simulink model "gm_uz_SVPWM_6ph"  (R2024a)
settings: Solver=FixedStepDiscrete  StartTime=0.0  StopTime=0.0004  RelTol=1e-3
undefined symbols (not defined in the file or in its folder): f_FPGA_clk, T_FPGA_clk
libraries: hdlsllib x7, simulink x1
(part 1 of 2)
settings Model: Creator=josef  LastModifiedBy=josef
settings SolverCC: AlgebraicLoopSolver=TrustRegion
settings DataIOCC: LimitDataPoints=on  SaveOutput=off  SaveTime=off
settings OptimizationCC: BlockReduction=off  ConditionallyExecuteInputs=off  DefaultParameterBehavior=Inlined  LifeSpan=inf
settings DebuggingCC: AlgebraicLoopMsg=error  InheritedTsInSrcMsg=none  SingleTaskRateTransMsg=error  UnconnectedInputMsg=warning  UnconnectedOutputMsg=warning  UnconnectedLineMsg=warning  AllowSymbolicDim=off  StrictBusMsg=ErrorOnBusTreatedAsVector  SFUnexpectedBacktrackingDiag=warning  SFNoUnconditionalDefaultTransitionDiag=warning  SFExecutionAtInitializationDiag=none  ArithmeticOperatorsInVariantConditions=warning
settings HardwareCC: ProdBitPerPointer=32  ProdBitPerSizeT=32  ProdBitPerPtrDiffT=32  ProdLargestAtomicFloat=None  ProdIntDivRoundTo=Undefined  ProdEndianess=Unspecified  ProdWordSize=32  ProdHWDeviceType=ASIC/FPGA->ASIC/FPGA  ProdEqTarget=off
settings ModelReferenceCC: EnableRefExpFcnMdlSchedulingChecks=on
settings SFSimCC: SimUseLocalCustomCode=off  CustomCodeUndefinedFunction=UseInterfaceOnly
settings RTWCC: RTWUseLocalCustomCode=off  GPUComputeCapability=3.5
settings CodeAppCC: StateflowObjectComments=on
settings GRTTargetCC: TargetLangStandard=C89/C90 (ANSI)
settings ConfigComp: CovScope=ReferencedModels  CovMetricSettings=dw  CovSaveCumulativeToWorkspaceVar=on  CovSaveSingleToWorkspaceVar=on  CovExternalEMLEnable=off  CovSFcnEnable=off

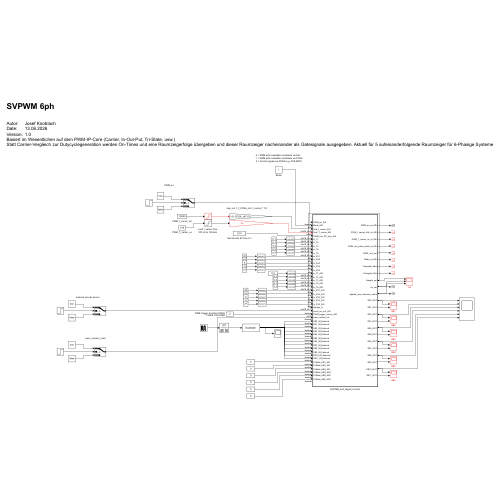
[thumbnail: Simulink's stored preview of the top-level diagram]
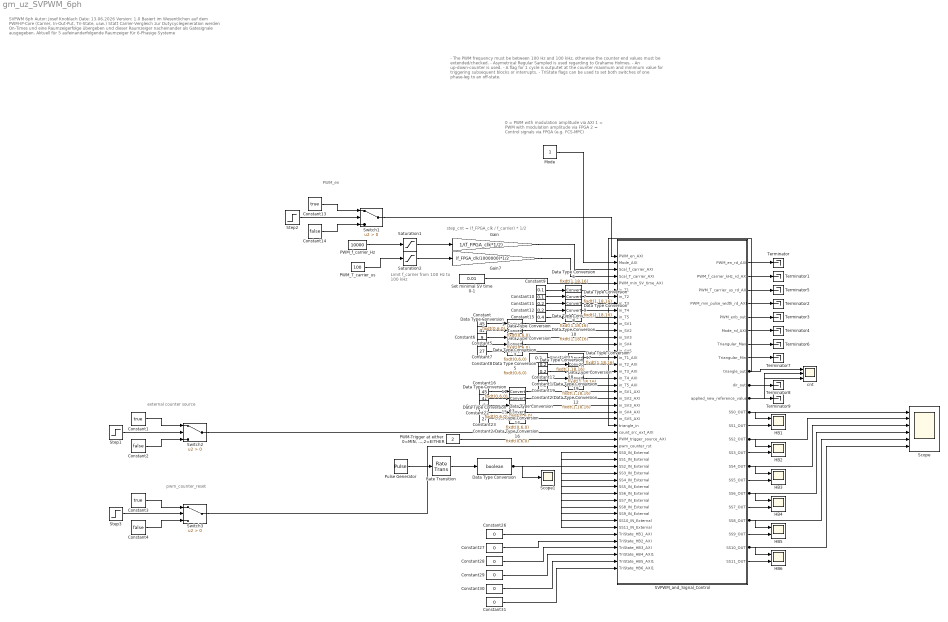
== system gm_uz_SVPWM_6ph ==
  note: pwm_counter_reset
  note: external counter source
  note: 0 = PWM with modulation amplitude via AXI
      | 1 = PWM with modulation amplitude via FPGA
      | 2 = Control signals via FPGA (e.g. FCS-MPC)
  note: step_cnt = (f_FPGA_clk / f_carrier) * 1/2
  note: SVPWM 6ph
      |
      | Autor: Josef Knoblach
      | Date: 13.06.2026
      | Version: 1.0
      | Basiert im Wesentlichen auf dem PWM-IP-Core (Carrier, In-Out-Put, Tri-State, usw.)
      | Statt Carrier-Vergleich zur Dutycyclegeneration werden On-Times und eine Raumzeigerfolge übergeben und dieser Raumzeiger nacheinander als Gatesignale ausgegeben. Aktuell für 5 aufeinanderfolgende Raumzeiger für 6-Phasige Systeme
  note: - The PWM frequency must be between 100 Hz and 100 kHz, otherwise the counter end values must be extended/checked.
      | - Asymetrical Regular Sampled is used regarding to Grahame Holmes.
      | - An up-down-counter is used.
      | - A flag for 1 cycle is outputet at the counter maximum and minimum value for triggering subsequent blocks or interrupts.
      | - TriState flags can be used to set both switches of one phase-leg to an off-state.
  note: Limit f_carrier from
      | 100 Hz to 100 kHz
  note: PWM_en
  Constant : Constant  Value=45  SampleTime=T_FPGA_clk
  Constant1 : Constant  Value=true  SampleTime=T_FPGA_clk
  Constant10 : Constant  Value=0.1  SampleTime=T_FPGA_clk
  Constant{11..12,17..18,20} (5 alike) : Constant  Value=0.2  SampleTime=T_FPGA_clk
  Constant13 : Constant  Value=true  SampleTime=T_FPGA_clk
  Constant14 : Constant  Value=false  SampleTime=T_FPGA_clk
  Constant15 : Constant  Value=0.4  SampleTime=T_FPGA_clk
  Constant16 : Constant  Value=45  SampleTime=T_FPGA_clk
  Constant19 : Constant  Value=0.1  SampleTime=T_FPGA_clk
  Constant2 : Constant  Value=false  SampleTime=T_FPGA_clk
  Constant21 : Constant  Value=41  SampleTime=T_FPGA_clk
  Constant22 : Constant  Value=9  SampleTime=T_FPGA_clk
  Constant23 : Constant  Value=11  SampleTime=T_FPGA_clk
  Constant24 : Constant  Value=27  SampleTime=T_FPGA_clk
  Constant25 : Constant  Value=0.3  SampleTime=T_FPGA_clk
  Constant{26..31} (6 alike) : Constant  Value=0  OutDataTypeStr=boolean  SampleTime=T_FPGA_clk
  Constant3 : Constant  Value=true  SampleTime=T_FPGA_clk
  Constant4 : Constant  Value=false  SampleTime=T_FPGA_clk
  Constant5 : Constant  Value=41  SampleTime=T_FPGA_clk
  Constant6 : Constant  Value=9  SampleTime=T_FPGA_clk
  Constant7 : Constant  Value=11  SampleTime=T_FPGA_clk
  Constant8 : Constant  Value=27  SampleTime=T_FPGA_clk
  Constant9 : Constant  Value=0.1  SampleTime=T_FPGA_clk
  Data Type Conversion : DataTypeConversion  OutDataTypeStr=boolean  SaturateOnIntegerOverflow=off  RndMeth=Floor
  Data Type Conversion{1..5,11,13..16} (10 alike) : DataTypeConversion  OutDataTypeStr=fixdt(0,6,0)  SaturateOnIntegerOverflow=off  RndMeth=Floor
  Data Type Conversion{6..10,12,17..20} (10 alike) : DataTypeConversion  OutDataTypeStr=fixdt(1,18,16)  SaturateOnIntegerOverflow=off  RndMeth=Floor
  Gain : Gain  Gain=1/(f_FPGA_clk*1/2)  OutDataTypeStr=fixdt(0,25,26)
  Gain7 : Gain  Gain=(f_FPGA_clk/1000000)*1/2  OutDataTypeStr=fixdt(0,25,0)
  HB{1..6} (6 alike) : Scope  NumInputPorts=2
  Mode : Constant  OutDataTypeStr=fixdt(0,2,0)  SampleTime=T_FPGA_clk
  "PWM-Trigger at either 0=MIN, 1=MAX,2=EITHER" : Constant  Value=2  OutDataTypeStr=uint32  SampleTime=T_FPGA_clk
  PWM_T_carrier_us : Constant  Value=100  OutDataTypeStr=uint32  SampleTime=T_FPGA_clk
  PWM_f_carrier_Hz : Constant  Value=10000  OutDataTypeStr=uint32  SampleTime=T_FPGA_clk
  Pulse Generator : DiscretePulseGenerator  PulseType=Time based  Period=0.0001  PulseWidth=5
  Rate Transition : RateTransition  OutPortSampleTime=T_FPGA_clk
  SVPWM_and_Signal_Control : Subsystem  TreatAsAtomicUnit=on
  Saturation1 : Saturate  UpperLimit=100000  LowerLimit=100
  Saturation2 : Saturate  UpperLimit=10000  LowerLimit=10
  Scope : Scope  NumInputPorts=6
  Scope1 : Scope
  Set minimal SV time 0-1 : Constant  Value=0.01  OutDataTypeStr=fixdt(1,18,16)  SampleTime=T_FPGA_clk
  Step1 : Step  Time=0.002  After=0  SampleTime=T_FPGA_clk
  Step2 : Step  Time=0.002  Before=1  SampleTime=T_FPGA_clk
  Step3 : Step  Time=0.00025  SampleTime=T_FPGA_clk
  Switch1 : Switch  Criteria=u2 > Threshold  SaturateOnIntegerOverflow=off  InputSameDT=off
  Switch2 : Switch  Criteria=u2 > Threshold  SaturateOnIntegerOverflow=off  InputSameDT=off
  Switch3 : Switch  Criteria=u2 > Threshold  SaturateOnIntegerOverflow=off  InputSameDT=off
  Terminator{,1..9} (10 alike) : Terminator
  cnt : Scope  NumInputPorts=3
  wires:
  SVPWM_and_Signal_Control/15(SS3_OUT) -> HB2/2
  SVPWM_and_Signal_Control/17(SS5_OUT) -> HB3/2
  SVPWM_and_Signal_Control/19(SS7_OUT) -> HB4/2
  SVPWM_and_Signal_Control/21(SS9_OUT) -> HB5/2
  SVPWM_and_Signal_Control/23(SS11_OUT) -> HB6/2
  SVPWM_and_Signal_Control/13(SS1_OUT) -> HB1/2
  SVPWM_and_Signal_Control/22(SS10_OUT) -> Scope/6, HB6/1
  SVPWM_and_Signal_Control/20(SS8_OUT) -> Scope/5, HB5/1
  SVPWM_and_Signal_Control/18(SS6_OUT) -> Scope/4, HB4/1
  SVPWM_and_Signal_Control/16(SS4_OUT) -> Scope/3, HB3/1
  SVPWM_and_Signal_Control/14(SS2_OUT) -> Scope/2, HB2/1
  SVPWM_and_Signal_Control/12(SS0_OUT) -> Scope/1, HB1/1
  Constant31/1 -> SVPWM_and_Signal_Control/47(TriState_HB6_AXI1)
  Constant30/1 -> SVPWM_and_Signal_Control/46(TriState_HB5_AXI1)
  Constant29/1 -> SVPWM_and_Signal_Control/45(TriState_HB4_AXI1)
  Constant28/1 -> SVPWM_and_Signal_Control/44(TriState_HB3_AXI)
  Constant27/1 -> SVPWM_and_Signal_Control/43(TriState_HB2_AXI)
  Constant26/1 -> SVPWM_and_Signal_Control/42(TriState_HB1_AXI)
  Data Type Conversion/1 -> SVPWM_and_Signal_Control/30(SS0_IN_External), SVPWM_and_Signal_Control/31(SS1_IN_External), SVPWM_and_Signal_Control/32(SS2_IN_External), SVPWM_and_Signal_Control/33(SS3_IN_External), SVPWM_and_Signal_Control/34(SS4_IN_External), SVPWM_and_Signal_Control/35(SS5_IN_External), SVPWM_and_Signal_Control/36(SS6_IN_External), SVPWM_and_Signal_Control/37(SS7_IN_External), SVPWM_and_Signal_Control/38(SS8_IN_External), SVPWM_and_Signal_Control/39(SS9_IN_External), SVPWM_and_Signal_Control/40(SS10_IN_External), SVPWM_and_Signal_Control/41(SS11_IN_External), Scope1/1
  Data Type Conversion16/1 -> SVPWM_and_Signal_Control/25(in_SV5_AXI)
  Data Type Conversion15/1 -> SVPWM_and_Signal_Control/24(in_SV4_AXI)
  Data Type Conversion14/1 -> SVPWM_and_Signal_Control/23(in_SV3_AXI)
  Data Type Conversion13/1 -> SVPWM_and_Signal_Control/22(in_SV2_AXI)
  Data Type Conversion11/1 -> SVPWM_and_Signal_Control/21(in_SV1_AXI)
  Constant16/1 -> Data Type Conversion11/1
  Constant24/1 -> Data Type Conversion16/1
  Constant23/1 -> Data Type Conversion15/1
  Constant22/1 -> Data Type Conversion14/1
  Constant21/1 -> Data Type Conversion13/1
  Constant17/1 -> Data Type Conversion18/1
  Constant18/1 -> Data Type Conversion19/1
  Constant19/1 -> Data Type Conversion20/1
  Constant20/1 -> Data Type Conversion12/1
  Constant25/1 -> Data Type Conversion17/1
  Data Type Conversion17/1 -> SVPWM_and_Signal_Control/16(in_T1_AXI)
  Data Type Conversion12/1 -> SVPWM_and_Signal_Control/20(in_T5_AXI)
  Data Type Conversion20/1 -> SVPWM_and_Signal_Control/19(in_T4_AXI)
  Data Type Conversion19/1 -> SVPWM_and_Signal_Control/18(in_T3_AXI)
  Data Type Conversion18/1 -> SVPWM_and_Signal_Control/17(in_T2_AXI)
  Data Type Conversion7/1 -> SVPWM_and_Signal_Control/7(in_T2)
  Data Type Conversion8/1 -> SVPWM_and_Signal_Control/8(in_T3)
  Data Type Conversion9/1 -> SVPWM_and_Signal_Control/9(in_T4)
  Data Type Conversion10/1 -> SVPWM_and_Signal_Control/10(in_T5)
  Data Type Conversion6/1 -> SVPWM_and_Signal_Control/6(in_T1)
  Constant9/1 -> Data Type Conversion6/1
  Constant15/1 -> Data Type Conversion10/1
  Constant12/1 -> Data Type Conversion9/1
  Constant11/1 -> Data Type Conversion8/1
  Constant10/1 -> Data Type Conversion7/1
  Constant5/1 -> Data Type Conversion2/1
  Constant6/1 -> Data Type Conversion3/1
  Constant7/1 -> Data Type Conversion4/1
  Constant8/1 -> Data Type Conversion5/1
  Constant/1 -> Data Type Conversion1/1
  Data Type Conversion1/1 -> SVPWM_and_Signal_Control/11(in_SV1)
  Data Type Conversion2/1 -> SVPWM_and_Signal_Control/12(in_SV2)
  Data Type Conversion3/1 -> SVPWM_and_Signal_Control/13(in_SV3)
  Data Type Conversion4/1 -> SVPWM_and_Signal_Control/14(in_SV4)
  Data Type Conversion5/1 -> SVPWM_and_Signal_Control/15(in_SV5)
  Constant13/1 -> Switch1/1
  PWM_f_carrier_Hz/1 -> Saturation1/1
  Mode/1 -> SVPWM_and_Signal_Control/2(Mode_AXI)
  Set minimal SV time 0-1/1 -> SVPWM_and_Signal_Control/5(PWM_min_SV_time_AXI)
  Step2/1 -> Switch1/2
  SVPWM_and_Signal_Control/8(Triangular_Min) -> Terminator7/1
  Gain/1 -> SVPWM_and_Signal_Control/3(Scal_f_carrier_AXI)
  SVPWM_and_Signal_Control/6(Mode_rd_AXI) -> Terminator4/1
  Gain7/1 -> SVPWM_and_Signal_Control/4(Scal_T_carrier_AXI)
  SVPWM_and_Signal_Control/5(PWM_enb_out) -> Terminator3/1
  SVPWM_and_Signal_Control/2(PWM_f_carrier_kHz_rd_AXI) -> Terminator1/1
  SVPWM_and_Signal_Control/7(Triangular_Max) -> Terminator6/1
  Constant1/1 -> Switch2/1
  SVPWM_and_Signal_Control/10(dir_out) -> Terminator8/1, cnt/2
  Constant14/1 -> Switch1/3
  Constant2/1 -> Switch2/3
  Saturation1/1 -> Gain/1
  Saturation2/1 -> Gain7/1
  Step1/1 -> Switch2/2
  PWM_T_carrier_us/1 -> Saturation2/1
  Rate Transition/1 -> Data Type Conversion/1
  SVPWM_and_Signal_Control/4(PWM_min_pulse_width_rd_AXI) -> Terminator2/1
  Switch2/1 -> SVPWM_and_Signal_Control/27(count_src_ext_AXI)
  Switch3/1 -> SVPWM_and_Signal_Control/29(pwm_counter_rst)
  SVPWM_and_Signal_Control/3(PWM_T_carrier_us_rd_AXI) -> Terminator5/1
  "PWM-Trigger at either 0=MIN, 1=MAX,2=EITHER"/1 -> SVPWM_and_Signal_Control/28(PWM_trigger_source_AXI)
  Step3/1 -> Switch3/2
  SVPWM_and_Signal_Control/1(PWM_en_rd_AXI) -> Terminator/1
  Switch1/1 -> SVPWM_and_Signal_Control/1(PWM_en_AXI)
  Constant4/1 -> Switch3/3
  SVPWM_and_Signal_Control/11(applied_new_reference_value) -> Terminator9/1, cnt/3
  Pulse Generator/1 -> Rate Transition/1
  Constant3/1 -> Switch3/1
  SVPWM_and_Signal_Control/9(triangle_out) -> cnt/1, SVPWM_and_Signal_Control/26(triangle_in)

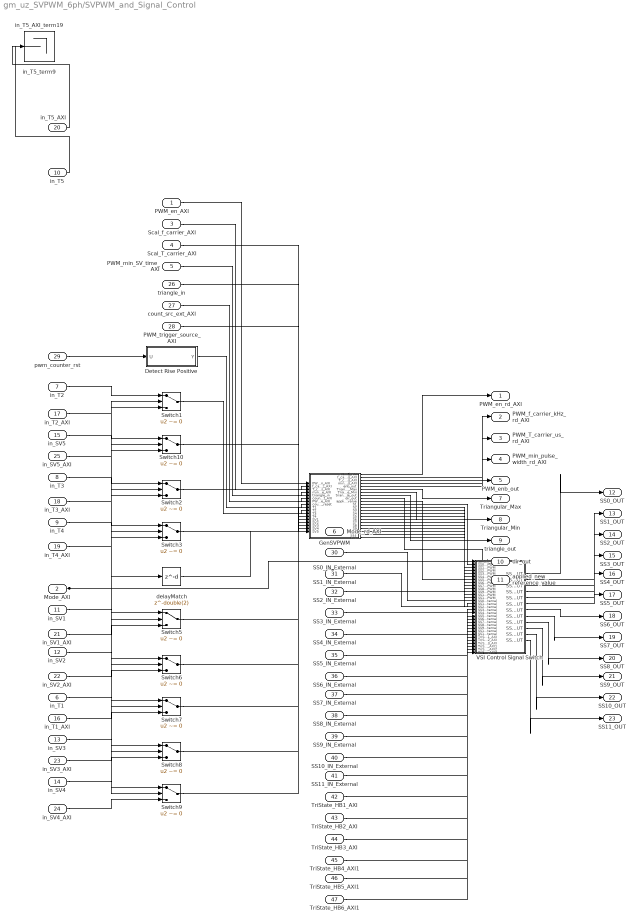
== system gm_uz_SVPWM_6ph/SVPWM_and_Signal_Control ==
  PWM_en_AXI : Inport  OutDataTypeStr=boolean  PortDimensions=1  SampleTime=1e-08
  Mode_AXI : Inport  Port=2  OutDataTypeStr=fixdt(0, 2, 0)  PortDimensions=1  SampleTime=1e-08
  Scal_f_carrier_AXI : Inport  Port=3  OutDataTypeStr=fixdt(0, 25, 26)  PortDimensions=1  SampleTime=1e-08
  Scal_T_carrier_AXI : Inport  Port=4  OutDataTypeStr=fixdt(0, 25, 0)  PortDimensions=1  SampleTime=1e-08
  PWM_min_SV_time_AXI : Inport  Port=5  OutDataTypeStr=fixdt(1, 18, 16)  PortDimensions=1  SampleTime=1e-08
  in_T1 : Inport  Port=6  OutDataTypeStr=fixdt(1, 18, 16)  PortDimensions=1  SampleTime=1e-08
  in_T2 : Inport  Port=7  OutDataTypeStr=fixdt(1, 18, 16)  PortDimensions=1  SampleTime=1e-08
  in_T3 : Inport  Port=8  OutDataTypeStr=fixdt(1, 18, 16)  PortDimensions=1  SampleTime=1e-08
  in_T4 : Inport  Port=9  OutDataTypeStr=fixdt(1, 18, 16)  PortDimensions=1  SampleTime=1e-08
  in_T5 : Inport  Port=10  OutDataTypeStr=fixdt(1, 18, 16)  PortDimensions=1  SampleTime=1e-08
  in_SV1 : Inport  Port=11  OutDataTypeStr=fixdt(0, 6, 0)  PortDimensions=1  SampleTime=1e-08
  in_SV2 : Inport  Port=12  OutDataTypeStr=fixdt(0, 6, 0)  PortDimensions=1  SampleTime=1e-08
  in_SV3 : Inport  Port=13  OutDataTypeStr=fixdt(0, 6, 0)  PortDimensions=1  SampleTime=1e-08
  in_SV4 : Inport  Port=14  OutDataTypeStr=fixdt(0, 6, 0)  PortDimensions=1  SampleTime=1e-08
  in_SV5 : Inport  Port=15  OutDataTypeStr=fixdt(0, 6, 0)  PortDimensions=1  SampleTime=1e-08
  in_T1_AXI : Inport  Port=16  OutDataTypeStr=fixdt(1, 18, 16)  PortDimensions=1  SampleTime=1e-08
  in_T2_AXI : Inport  Port=17  OutDataTypeStr=fixdt(1, 18, 16)  PortDimensions=1  SampleTime=1e-08
  in_T3_AXI : Inport  Port=18  OutDataTypeStr=fixdt(1, 18, 16)  PortDimensions=1  SampleTime=1e-08
  in_T4_AXI : Inport  Port=19  OutDataTypeStr=fixdt(1, 18, 16)  PortDimensions=1  SampleTime=1e-08
  in_T5_AXI : Inport  Port=20  OutDataTypeStr=fixdt(1, 18, 16)  PortDimensions=1  SampleTime=1e-08
  in_SV1_AXI : Inport  Port=21  OutDataTypeStr=fixdt(0, 6, 0)  PortDimensions=1  SampleTime=1e-08
  in_SV2_AXI : Inport  Port=22  OutDataTypeStr=fixdt(0, 6, 0)  PortDimensions=1  SampleTime=1e-08
  in_SV3_AXI : Inport  Port=23  OutDataTypeStr=fixdt(0, 6, 0)  PortDimensions=1  SampleTime=1e-08
  in_SV4_AXI : Inport  Port=24  OutDataTypeStr=fixdt(0, 6, 0)  PortDimensions=1  SampleTime=1e-08
  in_SV5_AXI : Inport  Port=25  OutDataTypeStr=fixdt(0, 6, 0)  PortDimensions=1  SampleTime=1e-08
  triangle_in : Inport  Port=26  OutDataTypeStr=fixdt(0, 18, 17)  PortDimensions=1  SampleTime=1e-08
  count_src_ext_AXI : Inport  Port=27  OutDataTypeStr=boolean  PortDimensions=1  SampleTime=1e-08
  PWM_trigger_source_AXI : Inport  Port=28  OutDataTypeStr=uint32  PortDimensions=1  SampleTime=1e-08
  pwm_counter_rst : Inport  Port=29  OutDataTypeStr=boolean  PortDimensions=1  SampleTime=1e-08
  SS0_IN_External : Inport  Port=30  OutDataTypeStr=boolean  PortDimensions=1  SampleTime=1e-08
  SS1_IN_External : Inport  Port=31  OutDataTypeStr=boolean  PortDimensions=1  SampleTime=1e-08
  SS2_IN_External : Inport  Port=32  OutDataTypeStr=boolean  PortDimensions=1  SampleTime=1e-08
  SS3_IN_External : Inport  Port=33  OutDataTypeStr=boolean  PortDimensions=1  SampleTime=1e-08
  SS4_IN_External : Inport  Port=34  OutDataTypeStr=boolean  PortDimensions=1  SampleTime=1e-08
  SS5_IN_External : Inport  Port=35  OutDataTypeStr=boolean  PortDimensions=1  SampleTime=1e-08
  SS6_IN_External : Inport  Port=36  OutDataTypeStr=boolean  PortDimensions=1  SampleTime=1e-08
  SS7_IN_External : Inport  Port=37  OutDataTypeStr=boolean  PortDimensions=1  SampleTime=1e-08
  SS8_IN_External : Inport  Port=38  OutDataTypeStr=boolean  PortDimensions=1  SampleTime=1e-08
  SS9_IN_External : Inport  Port=39  OutDataTypeStr=boolean  PortDimensions=1  SampleTime=1e-08
  SS10_IN_External : Inport  Port=40  OutDataTypeStr=boolean  PortDimensions=1  SampleTime=1e-08
  SS11_IN_External : Inport  Port=41  OutDataTypeStr=boolean  PortDimensions=1  SampleTime=1e-08
  TriState_HB1_AXI : Inport  Port=42  OutDataTypeStr=boolean  PortDimensions=1  SampleTime=1e-08
  TriState_HB2_AXI : Inport  Port=43  OutDataTypeStr=boolean  PortDimensions=1  SampleTime=1e-08
  TriState_HB3_AXI : Inport  Port=44  OutDataTypeStr=boolean  PortDimensions=1  SampleTime=1e-08
  TriState_HB4_AXI1 : Inport  Port=45  OutDataTypeStr=boolean  PortDimensions=1  SampleTime=1e-08
  TriState_HB5_AXI1 : Inport  Port=46  OutDataTypeStr=boolean  PortDimensions=1  SampleTime=1e-08
  TriState_HB6_AXI1 : Inport  Port=47  OutDataTypeStr=boolean  PortDimensions=1  SampleTime=1e-08
  Detect Rise Positive : Subsystem  mask(Detect Rise Positive){vinit=double(0), InputProcessing=Elements as channels (sample based), OutDataTypeStr=boolean}
      mask prompts: vinit "Simulink:masks:InitialCondition_MP"; InputProcessing "Simulink:masks:InputProcessing_MP"; OutDataTypeStr "Simulink:masks:OutputDataType_MP"
      mask help: Simulink:masks:DetectRisePositive_MD
      mask init:
      | InputProcessing = 'Elements as channels (sample based)';
      | OutDataTypeStr = 'boolean';
      | vinit = double(0);
      mask TypeOptions InputProcessing: Simulink:masks:ColumnsAsChannelsFrameBased | Simulink:masks:ElementsAsChannelsSampleBased
      mask TypeOptions OutDataTypeStr: Simulink:masks:uint8 | Simulink:masks:boolean
      mask Display: fprintf('U > 0\n&  NOT\nU/z > 0')
  GenSVPWM : Subsystem
  Switch{1..3,7} (4 alike) : Switch  Criteria=u2 ~= 0  Threshold=double(0)  OutDataTypeStr=fixdt(1, 18, 16)  SampleTime=1e-08  SaturateOnIntegerOverflow=off  InputSameDT=off
  Switch{5..6,8..10} (5 alike) : Switch  Criteria=u2 ~= 0  Threshold=double(0)  OutDataTypeStr=fixdt(0, 6, 0)  SampleTime=1e-08  SaturateOnIntegerOverflow=off  InputSameDT=off
  VSI Control Signal Switch : Subsystem
  delayMatch : Delay  DelayLength=double(2)  InitialCondition=0  SampleTime=1e-08
  in_T5_AXI_term19 : Terminator
  in_T5_term9 : Terminator
  PWM_en_rd_AXI : Outport  SampleTime=1e-08  VectorParamsAs1DForOutWhenUnconnected=off
  PWM_f_carrier_kHz_rd_AXI : Outport  Port=2  SampleTime=1e-08  VectorParamsAs1DForOutWhenUnconnected=off
  PWM_T_carrier_us_rd_AXI : Outport  Port=3  SampleTime=1e-08  VectorParamsAs1DForOutWhenUnconnected=off
  PWM_min_pulse_width_rd_AXI : Outport  Port=4  SampleTime=1e-08  VectorParamsAs1DForOutWhenUnconnected=off
  PWM_enb_out : Outport  Port=5  SampleTime=1e-08  VectorParamsAs1DForOutWhenUnconnected=off
  Mode_rd_AXI : Outport  Port=6  SampleTime=1e-08  VectorParamsAs1DForOutWhenUnconnected=off
  Triangular_Max : Outport  Port=7  SampleTime=1e-08  VectorParamsAs1DForOutWhenUnconnected=off
  Triangular_Min : Outport  Port=8  SampleTime=1e-08  VectorParamsAs1DForOutWhenUnconnected=off
  triangle_out : Outport  Port=9  SampleTime=1e-08  VectorParamsAs1DForOutWhenUnconnected=off
  dir_out : Outport  Port=10  SampleTime=1e-08  VectorParamsAs1DForOutWhenUnconnected=off
  applied_new_reference_value : Outport  Port=11  SampleTime=1e-08  VectorParamsAs1DForOutWhenUnconnected=off
  SS0_OUT : Outport  Port=12  SampleTime=1e-08  VectorParamsAs1DForOutWhenUnconnected=off
  SS1_OUT : Outport  Port=13  SampleTime=1e-08  VectorParamsAs1DForOutWhenUnconnected=off
  SS2_OUT : Outport  Port=14  SampleTime=1e-08  VectorParamsAs1DForOutWhenUnconnected=off
  SS3_OUT : Outport  Port=15  SampleTime=1e-08  VectorParamsAs1DForOutWhenUnconnected=off
  SS4_OUT : Outport  Port=16  SampleTime=1e-08  VectorParamsAs1DForOutWhenUnconnected=off
  SS5_OUT : Outport  Port=17  SampleTime=1e-08  VectorParamsAs1DForOutWhenUnconnected=off
  SS6_OUT : Outport  Port=18  SampleTime=1e-08  VectorParamsAs1DForOutWhenUnconnected=off
  SS7_OUT : Outport  Port=19  SampleTime=1e-08  VectorParamsAs1DForOutWhenUnconnected=off
  SS8_OUT : Outport  Port=20  SampleTime=1e-08  VectorParamsAs1DForOutWhenUnconnected=off
  SS9_OUT : Outport  Port=21  SampleTime=1e-08  VectorParamsAs1DForOutWhenUnconnected=off
  SS10_OUT : Outport  Port=22  SampleTime=1e-08  VectorParamsAs1DForOutWhenUnconnected=off
  SS11_OUT : Outport  Port=23  SampleTime=1e-08  VectorParamsAs1DForOutWhenUnconnected=off
  wires:
  PWM_en_AXI/1 -> GenSVPWM/1(PWM_en_AXI)
  delayMatch/1 -> Mode_rd_AXI/1
  Scal_f_carrier_AXI/1 -> GenSVPWM/2(f_carrier_kHz_AXI)
  Scal_T_carrier_AXI/1 -> GenSVPWM/3(T_carrier_us_AXI)
  PWM_min_SV_time_AXI/1 -> GenSVPWM/4(min_SV_time_AXI)
  in_T1/1 -> Switch7/1
  in_T2/1 -> Switch1/1
  in_T3/1 -> Switch2/1
  in_T4/1 -> Switch3/1
  in_T5/1 -> in_T5_term9/1
  in_SV1/1 -> Switch5/1
  in_SV2/1 -> Switch6/1
  in_SV3/1 -> Switch8/1
  in_SV4/1 -> Switch9/1
  in_SV5/1 -> Switch10/1
  in_T1_AXI/1 -> Switch7/3
  in_T2_AXI/1 -> Switch1/3
  in_T3_AXI/1 -> Switch2/3
  in_T4_AXI/1 -> Switch3/3
  in_T5_AXI/1 -> in_T5_AXI_term19/1
  in_SV1_AXI/1 -> Switch5/3
  in_SV2_AXI/1 -> Switch6/3
  in_SV3_AXI/1 -> Switch8/3
  in_SV4_AXI/1 -> Switch9/3
  in_SV5_AXI/1 -> Switch10/3
  triangle_in/1 -> GenSVPWM/5(triangle_in)
  count_src_ext_AXI/1 -> GenSVPWM/6(count_src_ext_AXI)
  PWM_trigger_source_AXI/1 -> GenSVPWM/7(PWM_trigger_source_AXI)
  pwm_counter_rst/1 -> Detect Rise Positive/1(U)
  SS0_IN_External/1 -> VSI Control Signal Switch/14(SS0_IN_External)
  SS1_IN_External/1 -> VSI Control Signal Switch/15(SS1_IN_External)
  SS2_IN_External/1 -> VSI Control Signal Switch/16(SS2_IN_External)
  SS3_IN_External/1 -> VSI Control Signal Switch/17(SS3_IN_External)
  SS4_IN_External/1 -> VSI Control Signal Switch/18(SS4_IN_External)
  SS5_IN_External/1 -> VSI Control Signal Switch/19(SS5_IN_External)
  SS6_IN_External/1 -> VSI Control Signal Switch/20(SS6_IN_External)
  SS7_IN_External/1 -> VSI Control Signal Switch/21(SS7_IN_External)
  SS8_IN_External/1 -> VSI Control Signal Switch/22(SS8_IN_External)
  SS9_IN_External/1 -> VSI Control Signal Switch/23(SS9_IN_External)
  SS10_IN_External/1 -> VSI Control Signal Switch/24(SS10_IN_External)
  SS11_IN_External/1 -> VSI Control Signal Switch/25(SS11_IN_External)
  TriState_HB1_AXI/1 -> VSI Control Signal Switch/26(TriState_HB1_AXI)
  TriState_HB2_AXI/1 -> VSI Control Signal Switch/27(TriState_HB2_AXI)
  TriState_HB3_AXI/1 -> VSI Control Signal Switch/28(TriState_HB3_AXI)
  TriState_HB4_AXI1/1 -> VSI Control Signal Switch/29(TriState_HB4_AXI1)
  TriState_HB5_AXI1/1 -> VSI Control Signal Switch/30(TriState_HB5_AXI2)
  TriState_HB6_AXI1/1 -> VSI Control Signal Switch/31(TriState_HB6_AXI3)
  Detect Rise Positive/1(Y) -> GenSVPWM/8(counter_reset)
  GenSVPWM/1(PWM_en_rd_AXI) -> PWM_en_rd_AXI/1
  GenSVPWM/2(f_carrier_kHz_rd_AXI) -> PWM_f_carrier_kHz_rd_AXI/1
  GenSVPWM/3(T_carrier_us_rd_AXI) -> PWM_T_carrier_us_rd_AXI/1
  GenSVPWM/4(min_SV_time_rd_AXI) -> PWM_min_pulse_width_rd_AXI/1
  GenSVPWM/5(enb_out) -> PWM_enb_out/1
  GenSVPWM/6(Triangle_Max) -> Triangular_Max/1
  GenSVPWM/7(Triangle_Min) -> Triangular_Min/1
  GenSVPWM/8(triangle_out) -> triangle_out/1
  GenSVPWM/9(dir_out) -> dir_out/1
  GenSVPWM/10(applied_new_reference_value) -> applied_new_reference_value/1
  GenSVPWM/11(S1) -> VSI Control Signal Switch/2(SS0_IN_PWM)
  GenSVPWM/12(S2) -> VSI Control Signal Switch/3(SS1_IN_PWM)
  GenSVPWM/13(S3) -> VSI Control Signal Switch/4(SS2_IN_PWM)
  GenSVPWM/14(S4) -> VSI Control Signal Switch/5(SS3_IN_PWM)
  GenSVPWM/15(S5) -> VSI Control Signal Switch/6(SS4_IN_PWM)
  GenSVPWM/16(S6) -> VSI Control Signal Switch/7(SS5_IN_PWM)
  GenSVPWM/17(S7) -> VSI Control Signal Switch/8(SS6_IN_PWM)
  GenSVPWM/18(S8) -> VSI Control Signal Switch/9(SS7_IN_PWM)
  GenSVPWM/19(S9) -> VSI Control Signal Switch/10(SS8_IN_PWM)
  GenSVPWM/20(S10) -> VSI Control Signal Switch/11(SS9_IN_PWM)
  GenSVPWM/21(S11) -> VSI Control Signal Switch/12(SS10_IN_PWM)
  GenSVPWM/22(S12) -> VSI Control Signal Switch/13(SS11_IN_PWM)
  Switch1/1 -> GenSVPWM/10(T2)
  Switch10/1 -> GenSVPWM/17(SV5)
  Switch2/1 -> GenSVPWM/11(T3)
  Switch3/1 -> GenSVPWM/12(T4)
  Switch5/1 -> GenSVPWM/13(SV1)
  Switch6/1 -> GenSVPWM/14(SV2)
  Switch7/1 -> GenSVPWM/9(T1)
  Switch8/1 -> GenSVPWM/15(SV3)
  Switch9/1 -> GenSVPWM/16(SV4)
  VSI Control Signal Switch/1(SS0_OUT) -> SS0_OUT/1
  VSI Control Signal Switch/2(SS1_OUT) -> SS1_OUT/1
  VSI Control Signal Switch/3(SS2_OUT) -> SS2_OUT/1
  VSI Control Signal Switch/4(SS3_OUT) -> SS3_OUT/1
  VSI Control Signal Switch/5(SS4_OUT) -> SS4_OUT/1
  VSI Control Signal Switch/6(SS5_OUT) -> SS5_OUT/1
  VSI Control Signal Switch/7(SS6_OUT) -> SS6_OUT/1
  VSI Control Signal Switch/8(SS7_OUT) -> SS7_OUT/1
  VSI Control Signal Switch/9(SS8_OUT) -> SS8_OUT/1
  VSI Control Signal Switch/10(SS9_OUT) -> SS9_OUT/1
  VSI Control Signal Switch/11(SS10_OUT) -> SS10_OUT/1
  VSI Control Signal Switch/12(SS11_OUT) -> SS11_OUT/1
  Mode_AXI/1 -> delayMatch/1, Switch9/2, Switch8/2, Switch7/2, Switch6/2, Switch5/2, Switch3/2, Switch2/2, Switch10/2, Switch1/2, VSI Control Signal Switch/1(Switch_AXI)

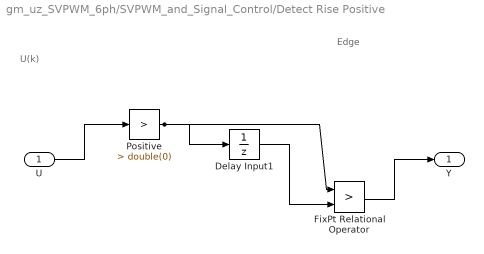
== system gm_uz_SVPWM_6ph/SVPWM_and_Signal_Control/Detect Rise Positive ==
  note: U(k)
  note: Edge
  U : Inport  OutDataTypeStr=boolean  SampleTime=1e-08
  Delay Input1 : UnitDelay  SampleTime=1e-08
  FixPt Relational Operator : RelationalOperator  Operator=>  OutDataTypeStr=boolean  SampleTime=1e-08  InputSameDT=off
  Positive : simulink/Logic and Bit Operations/Compare To Constant  relop=>  const=double(0)  OutDataTypeStr=boolean
  Y : Outport  SampleTime=1e-08
  wires:
  U/1 -> Positive/1
  Delay Input1/1 -> FixPt Relational Operator/2
  FixPt Relational Operator/1 -> Y/1
  Positive/1 -> FixPt Relational Operator/1, Delay Input1/1

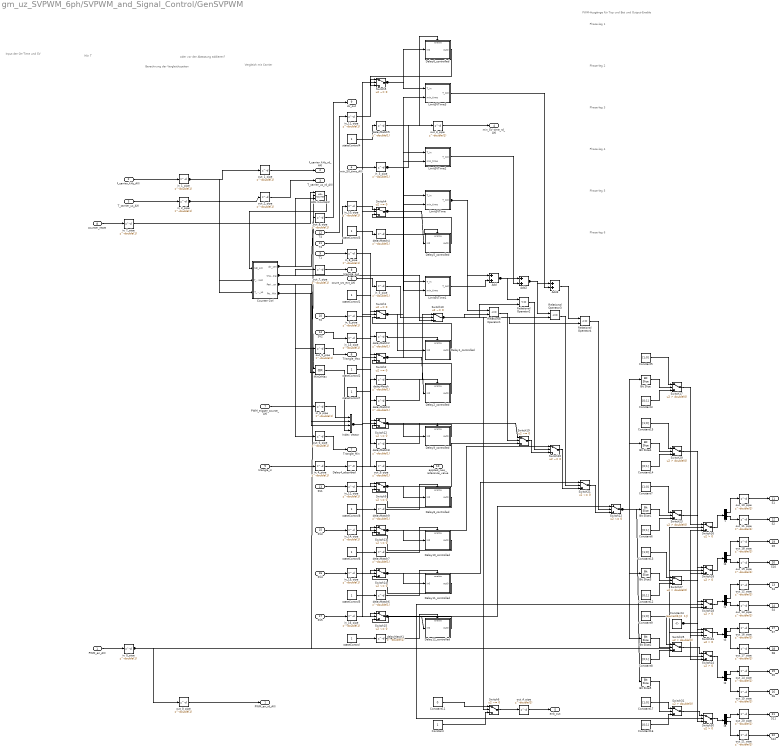
== system gm_uz_SVPWM_6ph/SVPWM_and_Signal_Control/GenSVPWM ==
  note: Phase-leg 6
  note: Phase-leg 5
  note: Phase-leg 4
  note: Phase-leg 3
  note: Phase-leg 2
  note: Phase-leg 1
  note: oder vor der Abtastung addieren?
  note: Input der On-Time und SV
  note: Berechnung der Vergleichszeiten
  note: Vergleich mit Carrier
  note: PWM-Ausgänge für Top und Bot und Output-Enable
  note: Min T
  PWM_en_AXI : Inport  OutDataTypeStr=boolean  PortDimensions=1  SampleTime=1e-08
  f_carrier_kHz_AXI : Inport  Port=2  OutDataTypeStr=fixdt(0, 25, 26)  PortDimensions=1  SampleTime=1e-08
  T_carrier_us_AXI : Inport  Port=3  OutDataTypeStr=fixdt(0, 25, 0)  PortDimensions=1  SampleTime=1e-08
  min_SV_time_AXI : Inport  Port=4  OutDataTypeStr=fixdt(1, 18, 16)  PortDimensions=1  SampleTime=1e-08
  triangle_in : Inport  Port=5  OutDataTypeStr=fixdt(0, 18, 17)  PortDimensions=1  SampleTime=1e-08
  count_src_ext_AXI : Inport  Port=6  OutDataTypeStr=boolean  PortDimensions=1  SampleTime=1e-08
  PWM_trigger_source_AXI : Inport  Port=7  OutDataTypeStr=uint32  PortDimensions=1  SampleTime=1e-08
  counter_reset : Inport  Port=8  OutDataTypeStr=boolean  PortDimensions=1  SampleTime=1e-08
  T1 : Inport  Port=9  OutDataTypeStr=fixdt(1, 18, 16)  PortDimensions=1  SampleTime=1e-08
  T2 : Inport  Port=10  OutDataTypeStr=fixdt(1, 18, 16)  PortDimensions=1  SampleTime=1e-08
  T3 : Inport  Port=11  OutDataTypeStr=fixdt(1, 18, 16)  PortDimensions=1  SampleTime=1e-08
  T4 : Inport  Port=12  OutDataTypeStr=fixdt(1, 18, 16)  PortDimensions=1  SampleTime=1e-08
  SV1 : Inport  Port=13  OutDataTypeStr=fixdt(0, 6, 0)  PortDimensions=1  SampleTime=1e-08
  SV2 : Inport  Port=14  OutDataTypeStr=fixdt(0, 6, 0)  PortDimensions=1  SampleTime=1e-08
  SV3 : Inport  Port=15  OutDataTypeStr=fixdt(0, 6, 0)  PortDimensions=1  SampleTime=1e-08
  SV4 : Inport  Port=16  OutDataTypeStr=fixdt(0, 6, 0)  PortDimensions=1  SampleTime=1e-08
  SV5 : Inport  Port=17  OutDataTypeStr=fixdt(0, 6, 0)  PortDimensions=1  SampleTime=1e-08
  Add : Sum  OutDataTypeStr=fixdt(1, 19, 16)  AccumDataTypeStr=fixdt(1, 19, 16)  SampleTime=1e-08
  Add2 : Sum  OutDataTypeStr=fixdt(1, 20, 16)  AccumDataTypeStr=fixdt(1, 20, 16)  SampleTime=1e-08
  Add3 : Sum  OutDataTypeStr=fixdt(1, 21, 16)  AccumDataTypeStr=fixdt(1, 21, 16)  SampleTime=1e-08
  Bit Slice : hdlsllib/Logic and Bit Operations/Bit Slice  lidx=double(0)  ridx=double(0)
  Bit Slice1 : hdlsllib/Logic and Bit Operations/Bit Slice  lidx=double(1)  ridx=double(1)
  Bit Slice2 : hdlsllib/Logic and Bit Operations/Bit Slice  lidx=double(2)  ridx=double(2)
  Bit Slice3 : hdlsllib/Logic and Bit Operations/Bit Slice  lidx=double(3)  ridx=double(3)
  Bit Slice4 : hdlsllib/Logic and Bit Operations/Bit Slice  lidx=double(4)  ridx=double(4)
  Bit Slice5 : hdlsllib/Logic and Bit Operations/Bit Slice  lidx=double(5)  ridx=double(5)
  Constant : Constant  OutDataTypeStr=boolean  SampleTime=1e-08
  Constant11 : Constant  Value=0  OutDataTypeStr=boolean  SampleTime=1e-08
  Constant{3,6,8,12,14,16} (6 alike) : Constant  Value=[0;1]  OutDataTypeStr=fixdt(0, 1, 0)  SampleTime=1e-08
  Constant{5,7,9,13,15,17} (6 alike) : Constant  Value=[1;0]  OutDataTypeStr=fixdt(0, 1, 0)  SampleTime=1e-08
  Constant4 : Constant  Value="repmat(0,[2  1])"  OutDataTypeStr=fixdt(0, 1, 0)  SampleTime=1e-08
  Counter Ctrl : Subsystem
  Delay10_controlled : Subsystem
  Delay11_controlled : Subsystem
  Delay12_controlled : Subsystem
  Delay1_controlled : Subsystem
  Delay2_controlled : Subsystem
  Delay4_absorbed : Delay  DelayLength=0
  Delay5_controlled : Subsystem
  Delay6_controlled : Subsystem
  Delay8_controlled : Subsystem
  Delay9_controlled : Subsystem
  HDL Counter2 : hdlsllib/Sources/HDL Counter  CountType=Free running  CountInit=0  CountStep=1  CountMax=100  CountFromType=Initial value  CountFrom=0  CountResetPort=on  CountLoadPort=off  CountEnbPort=on  CountDirPort=on  CountHitOutputPort=off  CountDataType=Unsigned  CountWordLen=20  CountFracLen=0  CountSampTime=1
  Index Vector : MultiPortSwitch  DataPortOrder=Zero-based contiguous  DiagnosticForDefault=None  zeroidx=on  SampleTime=1e-08  SaturateOnIntegerOverflow=off  InputSameDT=off
  LimitSVTime : Subsystem
  LimitSVTime1 : Subsystem
  LimitSVTime2 : Subsystem
  LimitSVTime3 : Subsystem
  MinOrMax : Logic  Operator=OR  AllPortsSameDT=off  OutDataTypeStr=boolean  SampleTime=1e-08
  Relational Operator{1..4} (4 alike) : RelationalOperator  Operator=<=  OutDataTypeStr=boolean  SampleTime=1e-08  InputSameDT=off
  Switch{1..2,4..5} (4 alike) : Switch  Criteria=u2 ~= 0  Threshold=double(0)  OutDataTypeStr=fixdt(1, 18, 16)  SampleTime=1e-08  SaturateOnIntegerOverflow=off  InputSameDT=off
  Switch10 : Switch  Criteria=u2 ~= 0  Threshold=double(0)  OutDataTypeStr=fixdt(0, 18, 17)  SampleTime=1e-08  SaturateOnIntegerOverflow=off  InputSameDT=off
  Switch{9,12..15,19..22} (9 alike) : Switch  Criteria=u2 ~= 0  Threshold=double(0)  OutDataTypeStr=fixdt(0, 6, 0)  SampleTime=1e-08  SaturateOnIntegerOverflow=off  InputSameDT=off
  Switch{16,18,24,26,28,30} (6 alike) : Switch  Criteria=u2 > Threshold  OutDataTypeStr=fixdt(0, 1, 0)  SampleTime=1e-08  SaturateOnIntegerOverflow=off  InputSameDT=off
  Switch{17,23,25,27,29,31} (6 alike) : Switch  Criteria=u2 > Threshold  Threshold=double(0)  OutDataTypeStr=fixdt(0, 1, 0)  SampleTime=1e-08  SaturateOnIntegerOverflow=off  InputSameDT=off
  Switch6 : Switch  Criteria=u2 ~= 0  Threshold=double(0)  OutDataTypeStr=boolean  SampleTime=1e-08  SaturateOnIntegerOverflow=off  InputSameDT=off
  delayMatch{,1..9} (10 alike) : Delay  DelayLength=double(1)  InitialCondition=0  SampleTime=1e-08
  in_0_pipe : Delay  DelayLength=double(1)  InitialCondition=0  SampleTime=1e-08
  in_10_pipe : Delay  DelayLength=double(1)  InitialCondition=0  SampleTime=1e-08
  in_11_pipe : Delay  DelayLength=double(1)  InitialCondition=0  SampleTime=1e-08
  in_12_pipe : Delay  DelayLength=double(1)  InitialCondition=0  SampleTime=1e-08
  in_13_pipe : Delay  DelayLength=double(1)  InitialCondition=0  SampleTime=1e-08
  in_14_pipe : Delay  DelayLength=double(1)  InitialCondition=0  SampleTime=1e-08
  in_15_pipe : Delay  DelayLength=double(1)  InitialCondition=0  SampleTime=1e-08
  in_16_pipe : Delay  DelayLength=double(1)  InitialCondition=0  SampleTime=1e-08
  in_1_pipe : Delay  DelayLength=double(1)  InitialCondition=0  SampleTime=1e-08
  in_2_pipe : Delay  DelayLength=double(1)  InitialCondition=0  SampleTime=1e-08
  in_3_pipe : Delay  DelayLength=double(1)  InitialCondition=0  SampleTime=1e-08
  in_4_pipe : Delay  DelayLength=double(1)  InitialCondition=0  SampleTime=1e-08
  in_5_pipe : Delay  DelayLength=double(1)  InitialCondition=0  SampleTime=1e-08
  in_6_pipe : Delay  DelayLength=double(1)  InitialCondition=0  SampleTime=1e-08
  in_7_pipe : Delay  DelayLength=double(1)  InitialCondition=0  SampleTime=1e-08
  in_8_pipe : Delay  DelayLength=double(1)  InitialCondition=0  SampleTime=1e-08
  in_9_pipe : Delay  DelayLength=double(1)  InitialCondition=0  SampleTime=1e-08
  out_0_pipe : Delay  DelayLength=double(1)  InitialCondition=0  SampleTime=1e-08
  out_10_pipe : Delay  DelayLength=double(1)  InitialCondition=0  SampleTime=1e-08
  out_11_pipe : Delay  DelayLength=double(1)  InitialCondition=0  SampleTime=1e-08
  out_12_pipe : Delay  DelayLength=double(1)  InitialCondition=0  SampleTime=1e-08
  out_13_pipe : Delay  DelayLength=double(1)  InitialCondition=0  SampleTime=1e-08
  out_14_pipe : Delay  DelayLength=double(1)  InitialCondition=0  SampleTime=1e-08
  out_15_pipe : Delay  DelayLength=double(1)  InitialCondition=0  SampleTime=1e-08
  out_16_pipe : Delay  DelayLength=double(1)  InitialCondition=0  SampleTime=1e-08
  out_17_pipe : Delay  DelayLength=double(1)  InitialCondition=0  SampleTime=1e-08
  out_18_pipe : Delay  DelayLength=double(1)  InitialCondition=0  SampleTime=1e-08
  out_19_pipe : Delay  DelayLength=double(1)  InitialCondition=0  SampleTime=1e-08
  out_1_pipe : Delay  DelayLength=double(1)  InitialCondition=0  SampleTime=1e-08
  out_20_pipe : Delay  DelayLength=double(1)  InitialCondition=0  SampleTime=1e-08
  out_21_pipe : Delay  DelayLength=double(1)  InitialCondition=0  SampleTime=1e-08
  out_2_pipe : Delay  DelayLength=double(1)  InitialCondition=0  SampleTime=1e-08
  out_3_pipe : Delay  DelayLength=double(1)  InitialCondition=0  SampleTime=1e-08
  out_4_pipe : Delay  DelayLength=double(1)  InitialCondition=0  SampleTime=1e-08
  out_5_pipe : Delay  DelayLength=double(1)  InitialCondition=0  SampleTime=1e-08
  out_6_pipe : Delay  DelayLength=double(1)  InitialCondition=0  SampleTime=1e-08
  out_7_pipe : Delay  DelayLength=double(1)  InitialCondition=0  SampleTime=1e-08
  out_8_pipe : Delay  DelayLength=double(1)  InitialCondition=0  SampleTime=1e-08
  out_9_pipe : Delay  DelayLength=double(1)  InitialCondition=0  SampleTime=1e-08
  stateControl{,1..8} (9 alike) : Constant  OutDataTypeStr=boolean  SampleTime=1e-08
  t{,1..5} (6 alike) : Demux  Outputs=2
  PWM_en_rd_AXI : Outport  SampleTime=1e-08  VectorParamsAs1DForOutWhenUnconnected=off
  f_carrier_kHz_rd_AXI : Outport  Port=2  SampleTime=1e-08  VectorParamsAs1DForOutWhenUnconnected=off
  T_carrier_us_rd_AXI : Outport  Port=3  SampleTime=1e-08  VectorParamsAs1DForOutWhenUnconnected=off
  min_SV_time_rd_AXI : Outport  Port=4  SampleTime=1e-08  VectorParamsAs1DForOutWhenUnconnected=off
  enb_out : Outport  Port=5  SampleTime=1e-08  VectorParamsAs1DForOutWhenUnconnected=off
  Triangle_Max : Outport  Port=6  SampleTime=1e-08  VectorParamsAs1DForOutWhenUnconnected=off
  Triangle_Min : Outport  Port=7  SampleTime=1e-08  VectorParamsAs1DForOutWhenUnconnected=off
  triangle_out : Outport  Port=8  SampleTime=1e-08  VectorParamsAs1DForOutWhenUnconnected=off
  dir_out : Outport  Port=9  SampleTime=1e-08  VectorParamsAs1DForOutWhenUnconnected=off
  applied_new_reference_value : Outport  Port=10  OutDataTypeStr=boolean  SampleTime=1e-08  VectorParamsAs1DForOutWhenUnconnected=off
  S1 : Outport  Port=11  SampleTime=1e-08  VectorParamsAs1DForOutWhenUnconnected=off
  S2 : Outport  Port=12  SampleTime=1e-08  VectorParamsAs1DForOutWhenUnconnected=off
  S3 : Outport  Port=13  SampleTime=1e-08  VectorParamsAs1DForOutWhenUnconnected=off
  S4 : Outport  Port=14  SampleTime=1e-08  VectorParamsAs1DForOutWhenUnconnected=off
  S5 : Outport  Port=15  SampleTime=1e-08  VectorParamsAs1DForOutWhenUnconnected=off
  S6 : Outport  Port=16  SampleTime=1e-08  VectorParamsAs1DForOutWhenUnconnected=off
  S7 : Outport  Port=17  SampleTime=1e-08  VectorParamsAs1DForOutWhenUnconnected=off
  S8 : Outport  Port=18  SampleTime=1e-08  VectorParamsAs1DForOutWhenUnconnected=off
  S9 : Outport  Port=19  SampleTime=1e-08  VectorParamsAs1DForOutWhenUnconnected=off
  S10 : Outport  Port=20  SampleTime=1e-08  VectorParamsAs1DForOutWhenUnconnected=off
  S11 : Outport  Port=21  SampleTime=1e-08  VectorParamsAs1DForOutWhenUnconnected=off
  S12 : Outport  Port=22  SampleTime=1e-08  VectorParamsAs1DForOutWhenUnconnected=off
  wires:
  in_0_pipe/1 -> Switch30/2, Switch28/2, Switch26/2, Switch24/2, Switch18/2, Switch16/2, out_0_pipe/1, HDL Counter2/2
  in_1_pipe/1 -> out_1_pipe/1, Counter Ctrl/2(f_carrier_kHz)
  in_2_pipe/1 -> out_2_pipe/1, Counter Ctrl/3(T_carrier_us)
  in_3_pipe/1 -> out_3_pipe/1, LimitSVTime1/2(min_time), LimitSVTime2/2(min_time), LimitSVTime3/2(min_time), LimitSVTime/2(min_time)
  in_5_pipe/1 -> Switch10/2
  in_6_pipe/1 -> Index Vector/1
  Add/1 -> Relational Operator2/1, Add2/1
  Add2/1 -> Relational Operator3/1, Add3/1
  Add3/1 -> Relational Operator4/1
  Bit Slice/1 -> Switch17/2
  Bit Slice1/1 -> Switch23/2
  Bit Slice2/1 -> Switch25/2
  Bit Slice3/1 -> Switch27/2
  Bit Slice4/1 -> Switch29/2
  Bit Slice5/1 -> Switch31/2
  Constant/1 -> Switch6/3
  Constant11/1 -> Switch6/1
  Constant12/1 -> Switch27/3
  Constant13/1 -> Switch27/1
  Constant14/1 -> Switch29/3
  Constant15/1 -> Switch29/1
  Constant16/1 -> Switch31/3
  Constant17/1 -> Switch31/1
  Constant3/1 -> Switch17/3
  Constant4/1 -> Switch30/3, Switch28/3, Switch26/3, Switch24/3, Switch18/3, Switch16/3
  Constant5/1 -> Switch17/1
  Constant6/1 -> Switch23/3
  Constant7/1 -> Switch23/1
  Constant8/1 -> Switch25/3
  Constant9/1 -> Switch25/1
  delayMatch/1 -> Switch10/1
  Index Vector/1 -> out_9_pipe/1, Switch15/2, Switch1/2, Switch2/2, Switch4/2, Switch5/2, Switch14/2, Switch13/2, Switch12/2, Switch9/2
  LimitSVTime/1(T_out) -> Relational Operator1/1, Add/1
  LimitSVTime1/1(T_out) -> Add/2
  LimitSVTime2/1(T_out) -> Add2/2
  LimitSVTime3/1(T_out) -> Add3/2
  MinOrMax/1 -> Index Vector/4
  Relational Operator1/1 -> Switch19/2
  Relational Operator2/1 -> Switch20/2
  Relational Operator3/1 -> Switch21/2
  Relational Operator4/1 -> Switch22/2
  Switch10/1 -> Switch6/2, Relational Operator4/2, Relational Operator3/2, Relational Operator2/2, Relational Operator1/2
  Switch16/1 -> t/1
  Switch17/1 -> Switch16/1
  Switch18/1 -> t1/1
  Switch19/1 -> Switch20/3
  Switch20/1 -> Switch21/3
  Switch21/1 -> Switch22/3
  Switch22/1 -> Bit Slice5/1, Bit Slice4/1, Bit Slice3/1, Bit Slice2/1, Bit Slice1/1, Bit Slice/1
  Switch23/1 -> Switch18/1
  Switch24/1 -> t2/1
  Switch25/1 -> Switch24/1
  Switch26/1 -> t3/1
  Switch27/1 -> Switch26/1
  Switch28/1 -> t4/1
  Switch29/1 -> Switch28/1
  Switch30/1 -> t5/1
  Switch31/1 -> Switch30/1
  Switch6/1 -> out_4_pipe/1
  out_0_pipe/1 -> PWM_en_rd_AXI/1
  out_1_pipe/1 -> f_carrier_kHz_rd_AXI/1
  out_2_pipe/1 -> T_carrier_us_rd_AXI/1
  out_3_pipe/1 -> min_SV_time_rd_AXI/1
  out_4_pipe/1 -> enb_out/1
  out_5_pipe/1 -> Triangle_Max/1
  out_6_pipe/1 -> Triangle_Min/1
  out_7_pipe/1 -> triangle_out/1
  out_8_pipe/1 -> dir_out/1
  out_9_pipe/1 -> applied_new_reference_value/1
  out_10_pipe/1 -> S1/1
  out_11_pipe/1 -> S2/1
  out_12_pipe/1 -> S3/1
  out_13_pipe/1 -> S4/1
  out_14_pipe/1 -> S5/1
  out_15_pipe/1 -> S6/1
  out_16_pipe/1 -> S7/1
  out_17_pipe/1 -> S8/1
  out_18_pipe/1 -> S9/1
  out_19_pipe/1 -> S10/1
  out_20_pipe/1 -> S11/1
  out_21_pipe/1 -> S12/1
  PWM_en_AXI/1 -> in_0_pipe/1
  f_carrier_kHz_AXI/1 -> in_1_pipe/1
  T_carrier_us_AXI/1 -> in_2_pipe/1
  min_SV_time_AXI/1 -> in_3_pipe/1
  triangle_in/1 -> in_4_pipe/1
  count_src_ext_AXI/1 -> in_5_pipe/1
  PWM_trigger_source_AXI/1 -> in_6_pipe/1
  counter_reset/1 -> in_7_pipe/1
  T1/1 -> in_8_pipe/1
  T2/1 -> in_9_pipe/1
  T3/1 -> in_10_pipe/1
  T4/1 -> in_11_pipe/1
  SV1/1 -> in_12_pipe/1
  SV2/1 -> in_13_pipe/1
  SV3/1 -> in_14_pipe/1
  SV4/1 -> in_15_pipe/1
  SV5/1 -> in_16_pipe/1
  t/1 -> out_10_pipe/1
  t/2 -> out_11_pipe/1
  t1/1 -> out_12_pipe/1
  t1/2 -> out_13_pipe/1
  t2/1 -> out_14_pipe/1
  t2/2 -> out_15_pipe/1
  t3/1 -> out_16_pipe/1
  t3/2 -> out_17_pipe/1
  t4/1 -> out_18_pipe/1
  t4/2 -> out_19_pipe/1
  t5/1 -> out_20_pipe/1
  t5/2 -> out_21_pipe/1
  Delay4_absorbed/1 -> delayMatch/1
  stateControl/1 -> delayMatch1/1
  stateControl1/1 -> delayMatch2/1
  stateControl2/1 -> delayMatch3/1
  stateControl3/1 -> delayMatch4/1
  stateControl4/1 -> delayMatch5/1
  stateControl5/1 -> delayMatch6/1
  stateControl6/1 -> delayMatch7/1
  stateControl7/1 -> delayMatch8/1
  stateControl8/1 -> delayMatch9/1
  Switch9/1 -> Delay8_controlled/1(in0), Switch19/3
  Delay8_controlled/1(out0) -> Switch9/3
  delayMatch9/1 -> Delay8_controlled/Enable
  in_12_pipe/1 -> Switch9/1
  Counter Ctrl/2(triangle_sig) -> Switch10/3, out_7_pipe/1
  Counter Ctrl/3(Period_CenterMax) -> MinOrMax/1, Index Vector/3, out_5_pipe/1
  Counter Ctrl/4(Period_CenterMin) -> MinOrMax/2, Index Vector/2, out_6_pipe/1
  Counter Ctrl/1(dir_ctrl) -> out_8_pipe/1, HDL Counter2/3
  in_7_pipe/1 -> HDL Counter2/1
  HDL Counter2/1 -> Counter Ctrl/1(hdl_cnt)
  Switch15/1 -> Delay12_controlled/1(in0), Switch22/1
  Delay12_controlled/1(out0) -> Switch15/3
  delayMatch1/1 -> Delay12_controlled/Enable
  in_16_pipe/1 -> Switch15/1
  Switch1/1 -> Delay1_controlled/1(in0), LimitSVTime/1(T_in)
  Delay1_controlled/1(out0) -> Switch1/3
  delayMatch2/1 -> Delay1_controlled/Enable
  in_8_pipe/1 -> Switch1/1
  Switch2/1 -> Delay2_controlled/1(in0), LimitSVTime1/1(T_in)
  Delay2_controlled/1(out0) -> Switch2/3
  delayMatch3/1 -> Delay2_controlled/Enable
  in_9_pipe/1 -> Switch2/1
  Switch4/1 -> Delay5_controlled/1(in0), LimitSVTime2/1(T_in)
  Delay5_controlled/1(out0) -> Switch4/3
  delayMatch4/1 -> Delay5_controlled/Enable
  in_10_pipe/1 -> Switch4/1
  Switch5/1 -> Delay6_controlled/1(in0), LimitSVTime3/1(T_in)
  Delay6_controlled/1(out0) -> Switch5/3
  delayMatch5/1 -> Delay6_controlled/Enable
  in_11_pipe/1 -> Switch5/1
  Switch14/1 -> Delay11_controlled/1(in0), Switch21/1
  Delay11_controlled/1(out0) -> Switch14/3
  delayMatch6/1 -> Delay11_controlled/Enable
  in_15_pipe/1 -> Switch14/1
  Switch13/1 -> Delay10_controlled/1(in0), Switch20/1
  Delay10_controlled/1(out0) -> Switch13/3
  delayMatch7/1 -> Delay10_controlled/Enable
  in_14_pipe/1 -> Switch13/1
  Switch12/1 -> Delay9_controlled/1(in0), Switch19/1
  Delay9_controlled/1(out0) -> Switch12/3
  delayMatch8/1 -> Delay9_controlled/Enable
  in_13_pipe/1 -> Switch12/1
  in_4_pipe/1 -> Delay4_absorbed/1
